simulink model "Final_7_Simulink"  (R2024b)
settings: Solver=ode45  StartTime=0.0  StopTime=tspan  RelTol=1e-3
values from neighbouring files (symbols this model uses):
  cap_omega_0 = [0; 0; 0]    [Final_7.m]
  E_b_ECI_0 = [phi_b_eci_0; theta_b_eci_0; psi_b_eci_0]    [Final_7.m]
  E_b_LVLH_0 = [phi_0; theta_0; psi_0]    [Final_7.m]
  I_s = 1.2    [Final_7.m]
  J_sc = I_tot    [Final_7.m]
  JD_0 = 2460390    [Final_7.m]
  k_d = 2 * zeta * w_n * I_tot    [Final_7.m]
  k_p = 2 * I_tot * w_n^2    [Final_7.m]
  m_b = [0; 0; -0.5]    [Final_7.m]
  q_b_ECI_0 = q_b_ECI_0(:)    [Final_7.m]
  q_b_LVLH_0 = [0; 0; 0; 1]    [Final_7.m]
  q_c = [0; 0; 0; 1]    [Final_7.m]
  sun_ECI = [1; 0; 0]    [Final_7.m]
  surfaceProperties = [n.sat.areas n.sat.rho n.sat.normal]    [Final_7.m]
  T_c = [0; 0; 0]    [Final_7.m]
  w_b_ECI_0 = [0.001; -0.001; 0.002]    [Final_7.m]
undefined symbols (not defined in the file or in its folder): r_ECI_0, v_ECI_0
settings Model: Creator=kedde  LastModifiedBy=kedde

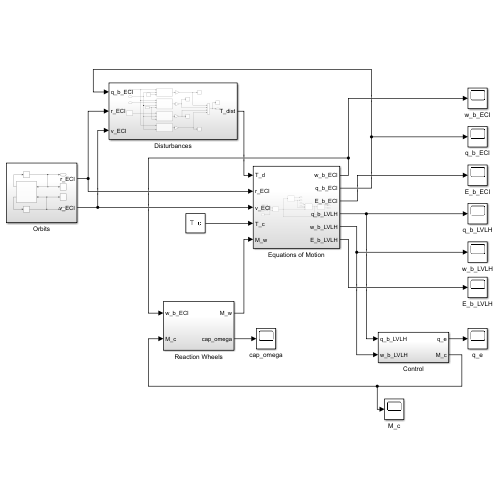
[thumbnail: Simulink's stored preview of the top-level diagram]
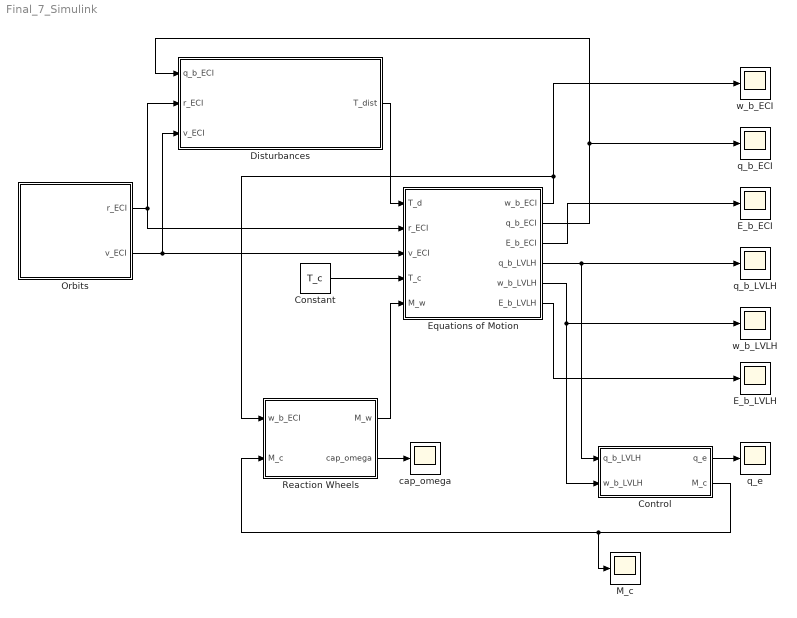
== system Final_7_Simulink ==
  Constant : Constant  Value=T_c
  Control : Subsystem
      settings: PortSchema="{\"entries\":[{\"content\":{\"sides\":[{\"content\":{\"connectorIds\":[\"Out1\",\"Out2\"]},\"type\":\"ConnectorPlacement.EquallySpacedRectSide\",\"uuid\":\"f6699d82-ad4a-4ee2-9e9e-65dce36df8d9\"},{\"content\":{\"connectorIds\":[\"In1\",\"In2\"],\"side\":\"RIGHT\"},\"type\":\"ConnectorPlacement.EquallySpacedRectSide\",\"uuid\":\"afcee84a-26e2-45dc-a34c-28f4183760c9\"},{\"content\":{\"side\":\"TOP\"},\"type\":\"ConnectorPlacement.EquallySpacedRectSide\",\"uuid\":\"e0497d07-e093-4203-954a-6559f552bf65\"},{\"content\":{\"side\":\"BOTTOM\"},\"type\":\"ConnectorPlacement.EquallySpacedRectSide\",\"uuid\":\"147dd8db-bb33-4af8-8890-1a9cf61198df\"}]},\"type\":\"ConnectorPlacement.EquallySpacedConnector\",\"uuid\":\"7d631ab2-7a88-49b1-aa1e-8fba77a3be9d\"}],\"packageUris\":[\"http://schema.mathworks.com/mf0/Connector/R2020b\"],\"version\":\"1.0\"}"
  Disturbances : Subsystem
  E_b_ECI : Scope
  E_b_LVLH : Scope
  Equations of Motion : Subsystem
  M_c : Scope
  Orbits : Subsystem
  Reaction Wheels : Subsystem
  cap_omega : Scope
  q_b_ECI : Scope
  q_b_LVLH : Scope
  q_e : Scope
  w_b_ECI : Scope
  w_b_LVLH : Scope
  wires:
  Orbits/2(v_ECI) -> Disturbances/3(v_ECI), Equations of Motion/3(v_ECI)
  Equations of Motion/6(E_b_LVLH) -> E_b_LVLH/1
  Orbits/1(r_ECI) -> Equations of Motion/2(r_ECI), Disturbances/2(r_ECI)
  Equations of Motion/5(w_b_LVLH) -> Control/2(w_b_LVLH), w_b_LVLH/1
  Equations of Motion/2(q_b_ECI) -> q_b_ECI/1, Disturbances/1(q_b_ECI)
  Constant/1 -> Equations of Motion/4(T_c)
  Equations of Motion/4(q_b_LVLH) -> q_b_LVLH/1, Control/1(q_b_LVLH)
  Equations of Motion/1(w_b_ECI) -> w_b_ECI/1, Reaction Wheels/1(w_b_ECI)
  Equations of Motion/3(E_b_ECI) -> E_b_ECI/1
  Disturbances/1(T_dist) -> Equations of Motion/1(T_d)
  Control/1(q_e) -> q_e/1
  Control/2(M_c) -> M_c/1, Reaction Wheels/2(M_c)
  Reaction Wheels/2(cap_omega) -> cap_omega/1
  Reaction Wheels/1(M_w) -> Equations of Motion/5(M_w)

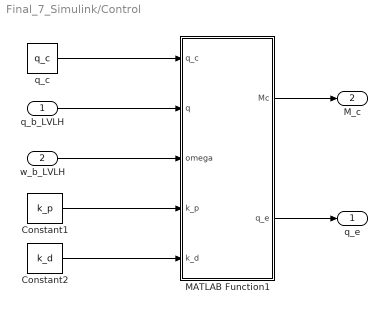
== system Final_7_Simulink/Control ==
  q_b_LVLH : Inport
  w_b_LVLH : Inport  Port=2  PortDimensions=[3 1]
  Constant1 : Constant  Value=k_p
  Constant2 : Constant  Value=k_d
  MATLAB Function1 : MATLAB Function  TreatAsAtomicUnit=on
  q_c : Constant  Value=q_c
  q_e : Outport
  M_c : Outport  Port=2  PortDimensions=[3 1]  VectorParamsAs1DForOutWhenUnconnected=off
  wires:
  Constant2/1 -> MATLAB Function1/5(k_d)
  w_b_LVLH/1 -> MATLAB Function1/3(omega)
  q_c/1 -> MATLAB Function1/1(q_c)
  MATLAB Function1/1(Mc) -> M_c/1
  q_b_LVLH/1 -> MATLAB Function1/2(q)
  Constant1/1 -> MATLAB Function1/4(k_p)
  MATLAB Function1/2(q_e) -> q_e/1

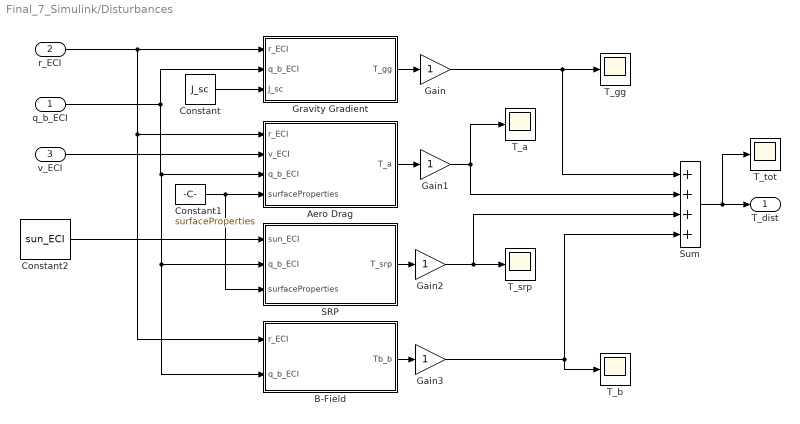
== system Final_7_Simulink/Disturbances ==
  q_b_ECI : Inport
  r_ECI : Inport  Port=2
  v_ECI : Inport  Port=3
  Aero Drag : MATLAB Function  TreatAsAtomicUnit=on
  B-Field : Subsystem
  Constant : Constant  Value=J_sc
  Constant1 : Constant  Value=surfaceProperties  VectorParams1D=off
  Constant2 : Constant  Value=sun_ECI
  Gain{,1..3} (4 alike) : Gain
  Gravity Gradient : MATLAB Function  TreatAsAtomicUnit=on
  SRP : MATLAB Function  TreatAsAtomicUnit=on
  Sum : Sum  Inputs=++++
  T_a : Scope
  T_b : Scope
  T_gg : Scope
  T_srp : Scope
  T_tot : Scope
  T_dist : Outport
  wires:
  Gain2/1 -> T_srp/1, Sum/3
  Aero Drag/1(T_a) -> Gain1/1
  Sum/1 -> T_tot/1, T_dist/1
  SRP/1(T_srp) -> Gain2/1
  v_ECI/1 -> Aero Drag/2(v_ECI)
  Gravity Gradient/1(T_gg) -> Gain/1
  Constant/1 -> Gravity Gradient/3(J_sc)
  Gain/1 -> Sum/1, T_gg/1
  Constant2/1 -> SRP/1(sun_ECI)
  Gain1/1 -> Sum/2, T_a/1
  q_b_ECI/1 -> B-Field/2(q_b_ECI), SRP/2(q_b_ECI), Aero Drag/3(q_b_ECI), Gravity Gradient/2(q_b_ECI)
  r_ECI/1 -> B-Field/1(r_ECI), Aero Drag/1(r_ECI), Gravity Gradient/1(r_ECI)
  B-Field/1(Tb_b) -> Gain3/1
  Constant1/1 -> SRP/3(surfaceProperties), Aero Drag/4(surfaceProperties)
  Gain3/1 -> T_b/1, Sum/4

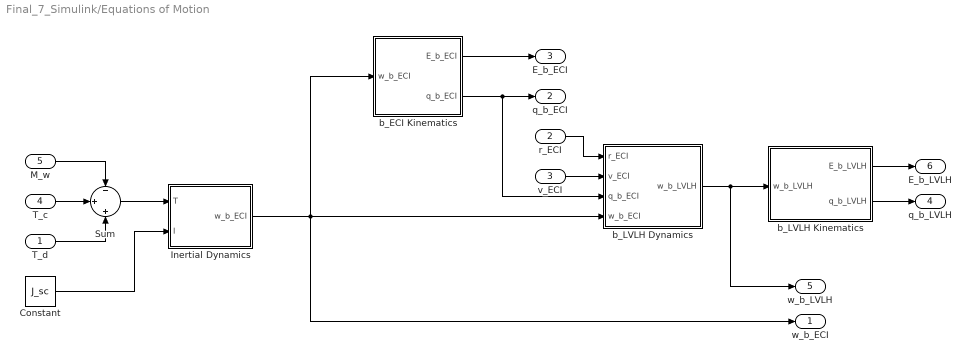
== system Final_7_Simulink/Equations of Motion ==
  T_d : Inport
  r_ECI : Inport  Port=2
  v_ECI : Inport  Port=3
  T_c : Inport  Port=4
  M_w : Inport  Port=5
  Constant : Constant  Value=J_sc
  Inertial Dynamics : Subsystem
  Sum : Sum  Inputs=-|+|+
  b_ECI Kinematics : Subsystem
  b_LVLH Dynamics : Subsystem
  b_LVLH Kinematics : Subsystem
  w_b_ECI : Outport  VectorParamsAs1DForOutWhenUnconnected=off
  q_b_ECI : Outport  Port=2  PortDimensions=[4 1]  VectorParamsAs1DForOutWhenUnconnected=off
  E_b_ECI : Outport  Port=3  PortDimensions=[3 1]  VectorParamsAs1DForOutWhenUnconnected=off
  q_b_LVLH : Outport  Port=4  PortDimensions=[4 1]  VectorParamsAs1DForOutWhenUnconnected=off
  w_b_LVLH : Outport  Port=5  PortDimensions=[3 1]  VectorParamsAs1DForOutWhenUnconnected=off
  E_b_LVLH : Outport  Port=6  PortDimensions=[3 1]  VectorParamsAs1DForOutWhenUnconnected=off
  wires:
  b_ECI Kinematics/1(E_b_ECI) -> E_b_ECI/1
  Constant/1 -> Inertial Dynamics/2(I)
  b_LVLH Kinematics/1(E_b_LVLH) -> E_b_LVLH/1
  Inertial Dynamics/1(w_b_ECI) -> w_b_ECI/1, b_LVLH Dynamics/4(w_b_ECI), b_ECI Kinematics/1(w_b_ECI)
  b_ECI Kinematics/2(q_b_ECI) -> b_LVLH Dynamics/3(q_b_ECI), q_b_ECI/1
  b_LVLH Kinematics/2(q_b_LVLH) -> q_b_LVLH/1
  r_ECI/1 -> b_LVLH Dynamics/1("r_ECI ")
  v_ECI/1 -> b_LVLH Dynamics/2(v_ECI)
  b_LVLH Dynamics/1(w_b_LVLH) -> w_b_LVLH/1, b_LVLH Kinematics/1(w_b_LVLH)
  T_d/1 -> Sum/3
  T_c/1 -> Sum/2
  Sum/1 -> Inertial Dynamics/1(T)
  M_w/1 -> Sum/1

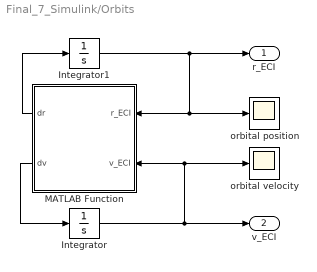
== system Final_7_Simulink/Orbits ==
  Integrator : Integrator  InitialCondition=v_ECI_0
  Integrator1 : Integrator  InitialCondition=r_ECI_0
  MATLAB Function : MATLAB Function  TreatAsAtomicUnit=on
  orbital position : Scope
  orbital velocity : Scope
  r_ECI : Outport  VectorParamsAs1DForOutWhenUnconnected=off
  v_ECI : Outport  Port=2  VectorParamsAs1DForOutWhenUnconnected=off
  wires:
  Integrator/1 -> orbital velocity/1, MATLAB Function/2(v_ECI), v_ECI/1
  Integrator1/1 -> orbital position/1, MATLAB Function/1(r_ECI), r_ECI/1
  MATLAB Function/1(dr) -> Integrator1/1
  MATLAB Function/2(dv) -> Integrator/1

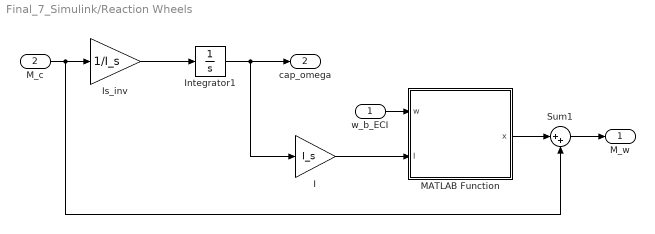
== system Final_7_Simulink/Reaction Wheels ==
  w_b_ECI : Inport
  M_c : Inport  Port=2
  I : Gain  Gain=I_s
  Integrator1 : Integrator  InitialCondition=cap_omega_0
  Is_inv : Gain  Gain=1/I_s
  MATLAB Function : MATLAB Function  TreatAsAtomicUnit=on
  Sum1 : Sum  Inputs=|++
  M_w : Outport
  cap_omega : Outport  Port=2
  wires:
  Integrator1/1 -> cap_omega/1, I/1
  Sum1/1 -> M_w/1
  w_b_ECI/1 -> MATLAB Function/1(w)
  I/1 -> MATLAB Function/2(I)
  Is_inv/1 -> Integrator1/1
  M_c/1 -> Is_inv/1, Sum1/2
  MATLAB Function/1(x) -> Sum1/1

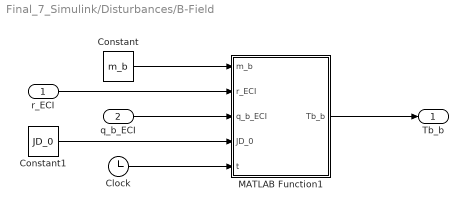
== system Final_7_Simulink/Disturbances/B-Field ==
  r_ECI : Inport
  q_b_ECI : Inport  Port=2
  Clock : Clock
  Constant : Constant  Value=m_b  VectorParams1D=off
  Constant1 : Constant  Value=JD_0
  MATLAB Function1 : MATLAB Function  TreatAsAtomicUnit=on
  Tb_b : Outport
  wires:
  MATLAB Function1/1(Tb_b) -> Tb_b/1
  q_b_ECI/1 -> MATLAB Function1/3(q_b_ECI)
  r_ECI/1 -> MATLAB Function1/2(r_ECI)
  Clock/1 -> MATLAB Function1/5(t)
  Constant1/1 -> MATLAB Function1/4(JD_0)
  Constant/1 -> MATLAB Function1/1(m_b)

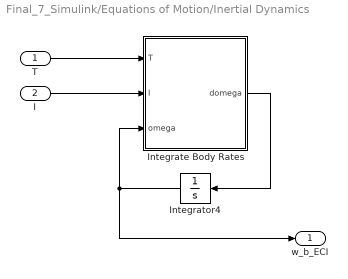
== system Final_7_Simulink/Equations of Motion/Inertial Dynamics ==
  T : Inport
  I : Inport  Port=2
  Integrate Body Rates : MATLAB Function  TreatAsAtomicUnit=on
  Integrator4 : Integrator  InitialCondition=w_b_ECI_0
  w_b_ECI : Outport  VectorParamsAs1DForOutWhenUnconnected=off
  wires:
  Integrate Body Rates/1(domega) -> Integrator4/1
  I/1 -> Integrate Body Rates/2(I)
  T/1 -> Integrate Body Rates/1(T)
  Integrator4/1 -> w_b_ECI/1, Integrate Body Rates/3(omega)

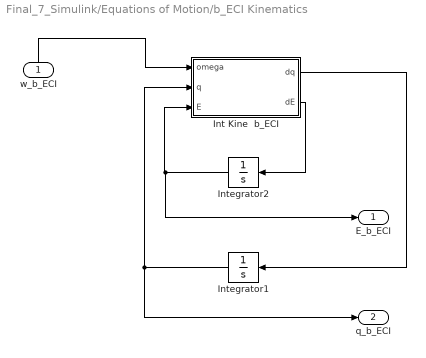
== system Final_7_Simulink/Equations of Motion/b_ECI Kinematics ==
  w_b_ECI : Inport
  Int Kine  b_ECI : MATLAB Function  TreatAsAtomicUnit=on
  Integrator1 : Integrator  InitialCondition=q_b_ECI_0
  Integrator2 : Integrator  InitialCondition=E_b_ECI_0
  E_b_ECI : Outport  PortDimensions=[3 1]  VectorParamsAs1DForOutWhenUnconnected=off
  q_b_ECI : Outport  Port=2  PortDimensions=[4 1]  VectorParamsAs1DForOutWhenUnconnected=off
  wires:
  w_b_ECI/1 -> Int Kine  b_ECI/1(omega)
  Int Kine  b_ECI/1(dq) -> Integrator1/1
  Int Kine  b_ECI/2(dE) -> Integrator2/1
  Integrator1/1 -> q_b_ECI/1, Int Kine  b_ECI/2(q)
  Integrator2/1 -> E_b_ECI/1, Int Kine  b_ECI/3(E)

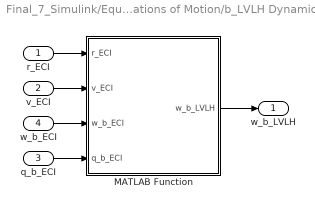
== system Final_7_Simulink/Equations of Motion/b_LVLH Dynamics ==
  "r_ECI " : Inport
  v_ECI : Inport  Port=2
  q_b_ECI : Inport  Port=3
  w_b_ECI : Inport  Port=4
  MATLAB Function : MATLAB Function  TreatAsAtomicUnit=on
  w_b_LVLH : Outport  VectorParamsAs1DForOutWhenUnconnected=off
  wires:
  MATLAB Function/1(w_b_LVLH) -> w_b_LVLH/1
  "r_ECI "/1 -> MATLAB Function/1(r_ECI)
  v_ECI/1 -> MATLAB Function/2(v_ECI)
  q_b_ECI/1 -> MATLAB Function/4(q_b_ECI)
  w_b_ECI/1 -> MATLAB Function/3(w_b_ECI)

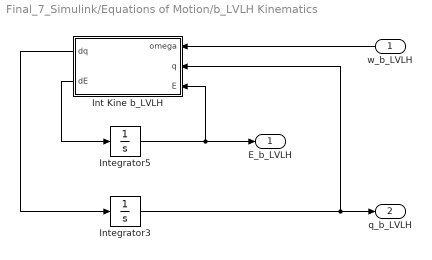
== system Final_7_Simulink/Equations of Motion/b_LVLH Kinematics ==
  w_b_LVLH : Inport
  Int Kine b_LVLH : MATLAB Function  TreatAsAtomicUnit=on
  Integrator3 : Integrator  InitialCondition=q_b_LVLH_0
  Integrator5 : Integrator  InitialCondition=E_b_LVLH_0
  E_b_LVLH : Outport  PortDimensions=[3 1]  VectorParamsAs1DForOutWhenUnconnected=off
  q_b_LVLH : Outport  Port=2  VectorParamsAs1DForOutWhenUnconnected=off
  wires:
  Int Kine b_LVLH/1(dq) -> Integrator3/1
  Integrator3/1 -> Int Kine b_LVLH/2(q), q_b_LVLH/1
  Int Kine b_LVLH/2(dE) -> Integrator5/1
  Integrator5/1 -> E_b_LVLH/1, Int Kine b_LVLH/3(E)
  w_b_LVLH/1 -> Int Kine b_LVLH/1(omega)

== matlab function Final_7_Simulink/Equations of Motion/b_LVLH Kinematics/Int Kine b_LVLH ==
  data: omega input; q input; dq output; E input; dE output
function [dq,dE] = kinematics(omega, q, E)
% ensure column vectors
omega = omega(:);
q = q(:);
E = E(:);

% unpack euler angles
phi = E(1);
theta = E(2);
psi = E(3);

% unpack quaternion
eps = q(1:3);
eta = q(4);

% derive euler angles
B = [1, sin(phi)*tan(theta), cos(phi)*tan(theta);
      0, cos(phi),           -sin(phi);
      0, sin(phi)/cos(theta), cos(phi)/cos(theta)];

dE = B * omega;

% derive quaternion
dq = zeros(4,1);
dq(1:3) = 0.5 * (eta*eye(3) + vect2cross(eps)) * omega;
dq(4) = -0.5 * eps' * omega;
end

function vect2cross = vect2cross(v)
    vect2cross = [ 0,   -v(3),  v(2)
                   v(3), 0,    -v(1)
                  -v(2), v(1),  0];
end

== matlab function Final_7_Simulink/Control/MATLAB Function1 ==
  data: q_c input; q input; omega input; k_p input; Mc output; k_d input; q_e output
function [Mc,q_e]  = control_law(q_c, q, omega, k_p, k_d)
%#codegen

q_e = quatMult(quatConjugate(q_c), q);
% q_e = quatMult(q, quatConjugate(q_c));
% Mc = -k_p * q_e(1:3,1) * sign(q_e(4)) - k_d*omega;
Mc = k_p * q_e(1:3,1) * sign(q_e(4)) + k_d*omega;

end

% ---------- OTHER NECESSARY FUNCTIONS ----------
function q_conj = quatConjugate(q)
% find the conjugate of a quaternion
% q(1:3) is eps
% q(4) is eta

    q_conj = [-q(1:3); q(4)];
end

function q_m = quatMult(q1, q2)
% multiply two quaternions q1 and q2
    v1 = q1(1:3);
    s1 = q1(4);

    v2 = q2(1:3);
    s2 = q2(4);
    
    v_out = s1*v2 + s2*v1 + cross(v1, v2);
    s_out = s1*s2 - dot(v1, v2);
    
    q_m = [v_out; s_out];

end

== matlab function Final_7_Simulink/Equations of Motion/Inertial Dynamics/Integrate Body Rates ==
  data: T input; I input; omega input; domega output
function domega = dynamics(T, I, omega)
% ensure column vectors
omega = omega(:);
T = T(:);

domega = I\(T - cross(omega, I*omega));
end

== matlab function Final_7_Simulink/Equations of Motion/b_ECI Kinematics/Int Kine  b_ECI ==
  data: omega input; q input; dq output; E input; dE output
function [dq, dE] = kinematics(omega, q, E)
% ensure column vectors
omega = omega(:);
q = q(:);
E = E(:);

% unpack euler angles
phi = E(1);
theta = E(2);
psi = E(3);

% unpack quaternions
eps = q(1:3);
eta = q(4);

% derive euler angles
B = [1, sin(phi)*tan(theta), cos(phi)*tan(theta);
      0, cos(phi),           -sin(phi);
      0, sin(phi)/cos(theta), cos(phi)/cos(theta)];

dE = B * omega;

% derive quaternion
dq = zeros(4,1);
dq(1:3) = 0.5 * (eta*eye(3) + vect2cross(eps)) * omega;
dq(4) = -0.5 * eps' * omega;
end


function vect2cross = vect2cross(v)
    vect2cross = [ 0,   -v(3),  v(2)
                   v(3), 0,    -v(1)
                  -v(2), v(1),  0];
end

== matlab function Final_7_Simulink/Disturbances/Gravity Gradient ==
  data: r_ECI input; T_gg output; q_b_ECI input; J_sc input
function T_gg = gg_torque(r_ECI, q_b_ECI, J_sc)
% Gravity-gradient torque in body coordinates
% Textbook model used:
%   Tg = (3*mu/r^5) * (r_b x (I*r_b))

    T_gg = zeros(3,1);

    % Earth gravitational parameter in SI [m^3/s^2]
    mu = 3.986004418e14;

    % Quaternion -> DCM, ECI to body
    q = q_b_ECI(:);
    e = q(1:3);
    eta = q(4);
    C_b_eci = (eta^2 - e.'*e)*eye(3) + 2*(e*e.') - 2*eta*vect2cross(e);

    % Convert r from km to m so units match J_sc [kg m^2]
    r_b = C_b_eci * (1000 * r_ECI(:));
    r   = norm(r_b);

    if r < 1e-12
        return
    end

    T_gg = -(3 * mu / r^5) * cross(r_b, J_sc * r_b);
    % T_gg = [0; 0; 0];
end

function C = vect2cross(v)
    C = [ 0    -v(3)  v(2);
          v(3)  0    -v(1);
         -v(2)  v(1)  0   ];
end

== matlab function Final_7_Simulink/Disturbances/Aero Drag ==
  data: r_ECI input; v_ECI input; T_a output; q_b_ECI input; surfaceProperties input
function T_a = aero_drag_torque(r_ECI, v_ECI, q_b_ECI, surfaceProperties)
T_a = zeros(3,1);
Cd = 2.5;

q   = q_b_ECI(:);
eps = q(1:3);
eta = q(4);
C_b_eci = (eta^2 - eps'*eps)*eye(3) + 2*(eps*eps') - 2*eta*vect2cross(eps);

v_b_m  = C_b_eci * v_ECI(:) * 1000;
v_mag  = norm(v_b_m);
v_unit = v_b_m / v_mag;

alt = norm(r_ECI) - 6378.137;
rho = atmospheric_density(alt);

for i = 1:size(surfaceProperties, 1)
    area   = surfaceProperties(i, 1);
    cp     = surfaceProperties(i, 2:4)';
    normal = surfaceProperties(i, 5:7)';
    % A_wet  = area * dot(normal, v_unit);
    A_wet  = -area * dot(normal, v_unit);
    if A_wet > 0
        F   = -(1/2) * rho * v_mag^2 * Cd * A_wet * v_unit;
        T_a = T_a + cross(cp, F);
    end
end
end

function C = vect2cross(v)
C = [ 0,   -v(3),  v(2);
      v(3),  0,   -v(1);
     -v(2),  v(1),  0  ];
end

function rho = atmospheric_density(alt)
    rho = 0.0;
    h0   = [0, 25, 30, 35, 40, 45, 50, 55, 60, 65, 70, 75, 80, 85, 90, ...
            95, 100, 110, 120, 130, 140, 150, 160, 180, 200, 250, 300, ...
            350, 400, 450, 500, 600, 700, 800, 900, 1000];
    rho0 = [1.225, 3.899e-2, 1.774e-2, 8.279e-3, 3.972e-3, 1.995e-3, ...
            1.057e-3, 5.821e-4, 3.206e-4, 1.718e-4, 8.770e-5, 4.178e-5, ...
            1.905e-5, 8.337e-6, 3.396e-6, 1.343e-6, 5.297e-7, 9.661e-8, ...
            2.438e-8, 8.484e-9, 3.845e-9, 2.070e-9, 1.224e-9, 5.464e-10, ...
            2.789e-10, 7.248e-11, 2.418e-11, 9.158e-12, 3.725e-12, ...
            1.585e-12, 6.967e-13, 1.454e-13, 3.614e-14, 1.170e-14, ...
            5.245e-15, 3.019e-15];
    H    = [8.44, 6.49, 6.75, 7.07, 7.47, 7.83, 7.95, 7.73, 7.29, 6.81, ...
            6.33, 6.00, 5.70, 5.41, 5.38, 5.74, 6.15, 8.06, 11.6, 16.1, ...
            20.6, 24.6, 26.3, 33.2, 38.5, 46.9, 52.5, 56.4, 59.4, 62.2, ...
            65.8, 79.0, 109.0, 164.0, 225.0, 268.0];

    idx = 1;  % default scalar
    for k = 1:length(h0)
        if alt >= h0(k)
            idx = k;
        end
    end

    rho = rho0(idx) * exp(-(alt - h0(idx)) / H(idx));
end

== matlab function Final_7_Simulink/Disturbances/SRP ==
  data: sun_ECI input; T_srp output; q_b_ECI input; surfaceProperties input
function T_srp = SRP_torque(sun_ECI, q_b_ECI, surfaceProperties)
% SRP torque in body coordinates
%
% Inputs:
%   sun_ECI           3x1 sun direction in ECI
%   q_b_ECI           4x1 quaternion [eps1; eps2; eps3; eta]
%   surfaceProperties Nx7 = [area, rho_x, rho_y, rho_z, n_x, n_y, n_z]
%
% Output:
%   T_srp             3x1 SRP torque in body frame [N m]
%
% Textbook model used:
%   total absorption
%   F_i = -p * A_i * max(n_i dot s_b, 0) * s_b
%   T_i = rho_i x F_i

    T_srp = zeros(3,1);

    % Solar radiation pressure near Earth [N/m^2]
    p = 4.5e-6;

    % Quaternion -> DCM, ECI to body
    q = q_b_ECI(:);
    e = q(1:3);
    eta = q(4);
    C_b_eci = (eta^2 - e.'*e)*eye(3) + 2*(e*e.') - 2*eta*vect2cross(e);

    % Sun direction in body frame
    s_b = -C_b_eci * sun_ECI(:);
    s_norm = norm(s_b);
    

    if s_norm < 1e-12
        return
    end

    s_hat = s_b / s_norm;

    % Loop over surfaces
    for i = 1:size(surfaceProperties,1)
        area   = surfaceProperties(i,1);
        rho_i  = surfaceProperties(i,2:4).';
        n_i    = surfaceProperties(i,5:7).';

        % illuminated if n dot s >= 0
        cos_alpha = dot(n_i, s_hat);

        if cos_alpha > 0
            F_i   = -p * area * cos_alpha * s_hat;
            T_srp = T_srp + cross(rho_i, F_i);
        end
    end
end

function C = vect2cross(v)
    C = [ 0    -v(3)  v(2);
          v(3)  0    -v(1);
         -v(2)  v(1)  0   ];
end

== matlab function Final_7_Simulink/Orbits/MATLAB Function ==
  data: r_ECI input; dr output; v_ECI input; dv output
function [dr,dv] = orbitalDynamics(r_ECI, v_ECI)

mu = 398600; % [km^3/s^2]
r_mag = norm(r_ECI);

dr = v_ECI; % [km/s]
dv = -(mu/r_mag^3) * r_ECI; % [km/s^2]
end

== matlab function Final_7_Simulink/Disturbances/B-Field/MATLAB Function1 ==
  data: m_b input; r_ECI input; q_b_ECI input; Tb_b output; JD_0 input; t input
function Tb_b = WMM(m_b, r_ECI, q_b_ECI, JD_0, t)

m_b = m_b(:);
r_ECI = r_ECI(:);
q_b_ECI = q_b_ECI(:);

% DGRF 2020 (given)
% a = 6371.2; %km
% g_11 = -1450.9; %nT
% h_11 = 4652.5; %nT
% g_10 = -29404.8; %nT
% m_ECEF = a^3*[g_11; h_11; g_10];

% converting given values to m and T
a = 6371.2 * 10^3;
g_11 = -1450.9 * 10^-9; 
h_11 = 4652.5 * 10^-9; 
g_10 = -29404.8 * 10^-9; 
m_ECEF = a^3*[g_11; h_11; g_10];

% local time is noon at initial given state, assuming t is in seconds
JD = JD_0 + t / 86400;

% first convert r from eci to ecef 

C_ecef_eci = eci2ecef(JD);

r_ECEF = C_ecef_eci * (1000 * r_ECI);

r = norm(r_ECEF);

B_ecef = (3 * (m_ECEF.' * r_ECEF) * r_ECEF - r^2 * m_ECEF) / r^5;

C_b_ECI = quat2C(q_b_ECI);

C_b_ecef = C_b_ECI * C_ecef_eci'; % doing successive rotions and transposing to get C_b_eci * C_eci_ecef

B_b = C_b_ecef * B_ecef;

Tb_b = vcross(m_b) * B_b;



    function C_ecef_eci = eci2ecef(JD) 
        T0 = (JD - 2451545) / 36525; 
        theta_G = mod(100.4606184 + 36000.77004*T0 + 0.000387933*T0^2 - 2.58*10^-8 * T0^3, 360); % in degs 
        theta_G = deg2rad(theta_G);
    
        C_ecef_eci = [cos(theta_G) sin(theta_G) 0
            -sin(theta_G) cos(theta_G) 0
            0 0 1]; % negative rotation about z axis 

    end 

        function vCross = vcross(v)
            vCross = [ 0,    -v(3),  v(2)
                      v(3),    0,   -v(1)
                     -v(2),   v(1),   0];
        end
        

        function C21 = quat2C(quaternion)
           
            epsilon = quaternion(1:3);
            eta = quaternion(4);
            I = [1 0 0
                0 1 0
                0 0 1];
            C21 = (2 * eta^2 - 1) * I + 2 * (epsilon * epsilon') - 2 * eta * vcross(epsilon);

        
        end

end

== matlab function Final_7_Simulink/Equations of Motion/b_LVLH Dynamics/MATLAB Function ==
  data: r_ECI input; v_ECI input; w_b_ECI input; q_b_ECI input; w_b_LVLH output
function w_b_LVLH = fcn(r_ECI, v_ECI, w_b_ECI, q_b_ECI)
% ensure column vectors
r_ECI = r_ECI(:);
v_ECI = v_ECI(:);
w_b_ECI = w_b_ECI(:);
q_b_ECI = q_b_ECI(:);

r_mag_sq = dot(r_ECI, r_ECI);

eps = q_b_ECI(1:3);
eta = q_b_ECI(4);

% angular velocity between LVLH and ECI
w_LVLH_ECI = cross(r_ECI, v_ECI) / r_mag_sq;

% rotation matrix body from ECI
C_b_ECI = (eta^2 - eps' * eps)*eye(3) + 2*(eps*eps') - 2*eta*vect2cross(eps);

% apply rotation matrix to angular velocity
w_b_LVLH = w_b_ECI - C_b_ECI*w_LVLH_ECI;
end

function vect2cross = vect2cross(v)
    vect2cross = [ 0,   -v(3),  v(2)
                   v(3), 0,    -v(1)
                  -v(2), v(1),  0];
end

== matlab function Final_7_Simulink/Reaction Wheels/MATLAB Function ==
  data: w input; x output; I input
function x = simplecross(w,I)

x = cross(w, I);
